simulink model "Adaptive_Cruise_Conrol_System"  (R2019a)
settings: Solver=VariableStepAuto  StartTime=0.0  StopTime=10.0  RelTol=1e-3
settings Model: Creator=賽維涅什  LastModifiedBy=賽維涅什

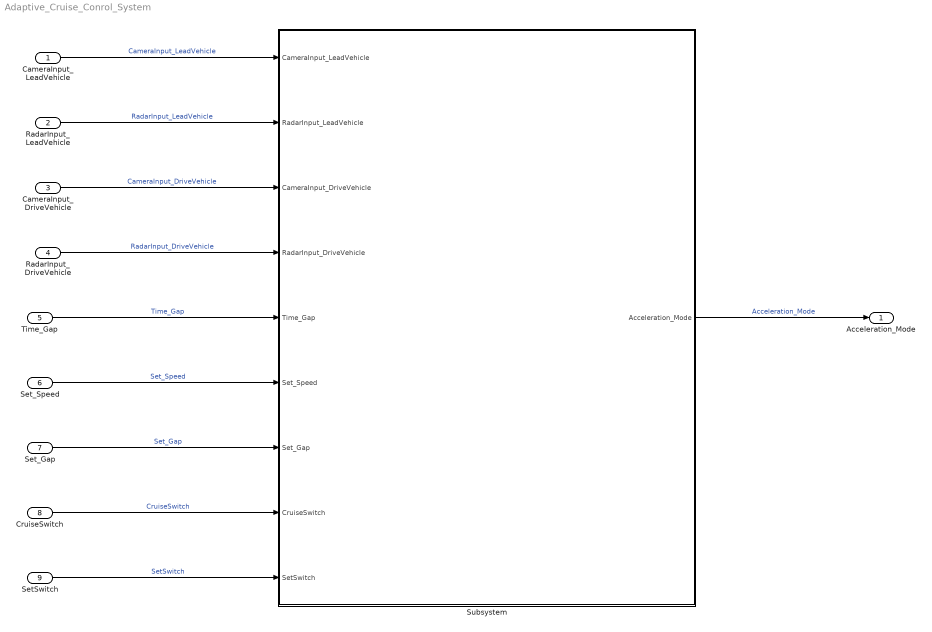
== system Adaptive_Cruise_Conrol_System ==
  CameraInput_LeadVehicle : Inport
  RadarInput_LeadVehicle : Inport  Port=2
  CameraInput_DriveVehicle : Inport  Port=3
  RadarInput_DriveVehicle : Inport  Port=4
  Time_Gap : Inport  Port=5
  Set_Speed : Inport  Port=6
  Set_Gap : Inport  Port=7
  CruiseSwitch : Inport  Port=8
  SetSwitch : Inport  Port=9
  Subsystem : Subsystem
  Acceleration_Mode : Outport
  wires:
  CameraInput_LeadVehicle/1 -> Subsystem/1(CameraInput_LeadVehicle)  "CameraInput_LeadVehicle"
  RadarInput_LeadVehicle/1 -> Subsystem/2(RadarInput_LeadVehicle)  "RadarInput_LeadVehicle"
  CameraInput_DriveVehicle/1 -> Subsystem/3(CameraInput_DriveVehicle)  "CameraInput_DriveVehicle"
  RadarInput_DriveVehicle/1 -> Subsystem/4(RadarInput_DriveVehicle)  "RadarInput_DriveVehicle"
  Time_Gap/1 -> Subsystem/5(Time_Gap)  "Time_Gap"
  Set_Speed/1 -> Subsystem/6(Set_Speed)  "Set_Speed"
  Set_Gap/1 -> Subsystem/7(Set_Gap)  "Set_Gap"
  CruiseSwitch/1 -> Subsystem/8(CruiseSwitch)  "CruiseSwitch"
  SetSwitch/1 -> Subsystem/9(SetSwitch)  "SetSwitch"
  Subsystem/1(Acceleration_Mode) -> Acceleration_Mode/1  "Acceleration_Mode"

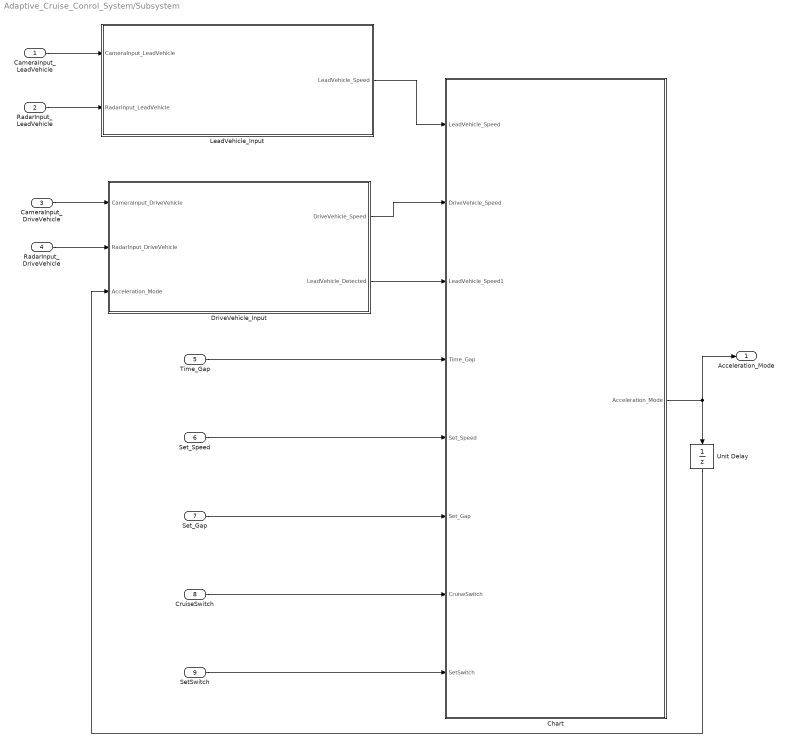
== system Adaptive_Cruise_Conrol_System/Subsystem ==
  CameraInput_LeadVehicle : Inport
  RadarInput_LeadVehicle : Inport  Port=2
  CameraInput_DriveVehicle : Inport  Port=3
  RadarInput_DriveVehicle : Inport  Port=4
  Time_Gap : Inport  Port=5
  Set_Speed : Inport  Port=6
  Set_Gap : Inport  Port=7
  CruiseSwitch : Inport  Port=8
  SetSwitch : Inport  Port=9
  Chart : Stateflow chart  BlockKeywords=__PRM__SERIALIZED__DATA__:Stateflow Chart,Stateflow Diagram  TreatAsAtomicUnit=on
  DriveVehicle_Input : Subsystem
  LeadVehicle_Input : Subsystem
  Unit Delay : UnitDelay  SampleTime=-1  HasFrameUpgradeWarning=on
  Acceleration_Mode : Outport
  wires:
  CameraInput_LeadVehicle/1 -> LeadVehicle_Input/1(CameraInput_LeadVehicle)
  DriveVehicle_Input/1(DriveVehicle_Speed) -> Chart/2(DriveVehicle_Speed)
  Chart/1(Acceleration_Mode) -> Acceleration_Mode/1, Unit Delay/1
  RadarInput_LeadVehicle/1 -> LeadVehicle_Input/2(RadarInput_LeadVehicle)
  Set_Speed/1 -> Chart/5(Set_Speed)
  Set_Gap/1 -> Chart/6(Set_Gap)
  CameraInput_DriveVehicle/1 -> DriveVehicle_Input/1(CameraInput_DriveVehicle)
  LeadVehicle_Input/1(LeadVehicle_Speed) -> Chart/1(LeadVehicle_Speed)
  Unit Delay/1 -> DriveVehicle_Input/3(Acceleration_Mode)
  CruiseSwitch/1 -> Chart/7(CruiseSwitch)
  Time_Gap/1 -> Chart/4(Time_Gap)
  DriveVehicle_Input/2(LeadVehicle_Detected) -> Chart/3(LeadVehicle_Speed1)
  RadarInput_DriveVehicle/1 -> DriveVehicle_Input/2(RadarInput_DriveVehicle)
  SetSwitch/1 -> Chart/8(SetSwitch)

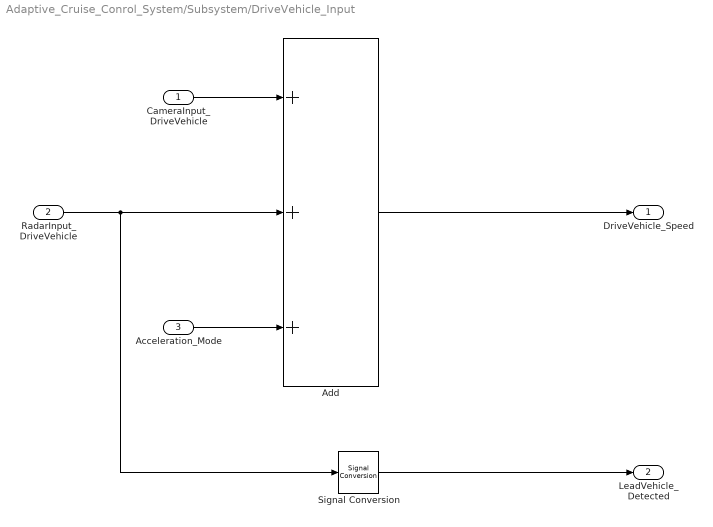
== system Adaptive_Cruise_Conrol_System/Subsystem/DriveVehicle_Input ==
  CameraInput_DriveVehicle : Inport
  RadarInput_DriveVehicle : Inport  Port=2
  Acceleration_Mode : Inport  Port=3
  Add : Sum  Inputs=+++
  Signal Conversion : SignalConversion  OverrideOpt=off
  DriveVehicle_Speed : Outport
  LeadVehicle_Detected : Outport  Port=2
  wires:
  CameraInput_DriveVehicle/1 -> Add/1
  RadarInput_DriveVehicle/1 -> Signal Conversion/1, Add/2
  Acceleration_Mode/1 -> Add/3
  Add/1 -> DriveVehicle_Speed/1
  Signal Conversion/1 -> LeadVehicle_Detected/1

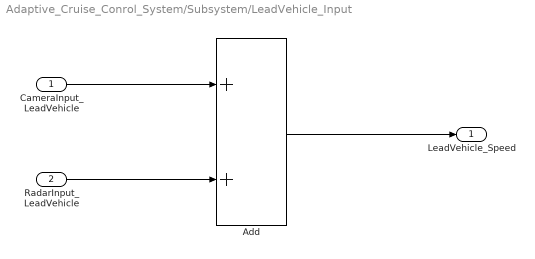
== system Adaptive_Cruise_Conrol_System/Subsystem/LeadVehicle_Input ==
  CameraInput_LeadVehicle : Inport
  RadarInput_LeadVehicle : Inport  Port=2
  Add : Sum
  LeadVehicle_Speed : Outport
  wires:
  CameraInput_LeadVehicle/1 -> Add/1
  RadarInput_LeadVehicle/1 -> Add/2
  Add/1 -> LeadVehicle_Speed/1

== stateflow chart Adaptive_Cruise_Conrol_System/Subsystem/Chart ==
  state ACC_ON_MODE
    en:Acceleration_Mode=1;
    state LeadVehicle_Detected_Follow
      en: Acceleration_Mode = 2;
    state LeadVehicle_Detected_Resume
      en: Acceleration_Mode = 3;
    state LeadVehicle_Not_Detected
      en: Acceleration_Mode = 1;
    state LeadVehicle_Speed_lessthan_set_Speed
      en: Acceleration_Mode = 4;
    state LeadVehicle_Not_Detected_Resume
      en: Acceleration_Mode = 1;
    state LeadVehicle_Speed_equal_Set_Speed
      en: Acceleration_Mode = 5;
    (default) -> LeadVehicle_Detected_Follow
    LeadVehicle_Detected_Follow -> LeadVehicle_Not_Detected [order 1] : [LeadVehicle_Detected == 0]
    LeadVehicle_Detected_Resume -> LeadVehicle_Detected_Follow [order 1] : [(DriveVehicle_Speed == Set_Speed)&&...
        | (LeadVehicle_Speed >= Set_Speed) &&...
        | (Time_Gap>= Set_Gap)]
    LeadVehicle_Detected_Resume -> LeadVehicle_Speed_equal_Set_Speed [order 2] : [(DriveVehicle_Speed<Set_Speed)&&...
        | (LeadVehicle_Speed > DriveVehicle_Speed)&&...
        | (Time_Gap >= Set_Gap)]
    LeadVehicle_Not_Detected -> LeadVehicle_Detected_Follow [order 1] : [(LeadVehicle_Detected == 1) &&...
        |  (DriveVehicle_Speed == Set_Speed) &&...
        | (LeadVehicle_Speed >= Set_Speed)&&...
        | (Time_Gap >= Set_Gap)]
    LeadVehicle_Speed_equal_Set_Speed -> LeadVehicle_Detected_Resume [order 2] : [(DriveVehicle_Speed<Set_Speed)&&...
        | (LeadVehicle_Speed>DriveVehicle_Speed)||...
        | (Time_Gap>=Set_Gap)]
    LeadVehicle_Detected_Follow -> LeadVehicle_Speed_lessthan_set_Speed [order 2] : [(LeadVehicle_Detected == 1) && ...
        | (LeadVehicle_Speed < Set_Speed)||...
        |  (Time_Gap< Set_Gap)]
    LeadVehicle_Not_Detected -> LeadVehicle_Speed_lessthan_set_Speed [order 2] : [(LeadVehicle_Detected == 1) &&...
        | (LeadVehicle_Speed < Set_Speed)||...
        | (Time_Gap < Set_Gap)]
    LeadVehicle_Speed_lessthan_set_Speed -> LeadVehicle_Not_Detected [order 1] : [(LeadVehicle_Detected == 0)&&...
        | (DriveVehicle_Speed == Set_Speed)]
    LeadVehicle_Speed_equal_Set_Speed -> LeadVehicle_Speed_lessthan_set_Speed [order 3] : [(LeadVehicle_Speed<Set_Speed)&&...
        | (LeadVehicle_Speed<DriveVehicle_Speed)||...
        | (Time_Gap==0.75*Set_Gap)]
    LeadVehicle_Speed_lessthan_set_Speed -> LeadVehicle_Speed_equal_Set_Speed [order 2] : [((LeadVehicle_Speed*1.25>=DriveVehicle_Speed)&&...
        | (LeadVehicle_Speed*0.75<=DriveVehicle_Speed))&&...
        | (DriveVehicle_Speed<Set_Speed)&&...
        | ((Time_Gap<=1.25*Set_Gap)&&...
        | (Time_Gap>=0.75*Set_Gap))]
    LeadVehicle_Speed_equal_Set_Speed -> LeadVehicle_Not_Detected_Resume [order 1] : [(LeadVehicle_Detected == 0)||...
        | (DriveVehicle_Speed <= Set_Speed)]
  state ACC_OFF_MODE
    en: Acceleration_Mode=0;
  state ACC_STANDBY_MODE
    en: Acceleration_Mode=1;
  (default) -> ACC_OFF_MODE
  ACC_ON_MODE -> ACC_OFF_MODE [order 2] : [CruiseSwitch==0]
  ACC_STANDBY_MODE -> ACC_OFF_MODE [order 2] : [CruiseSwitch == 0]
  ACC_OFF_MODE -> ACC_STANDBY_MODE : [CruiseSwitch == 1]
  ACC_ON_MODE -> ACC_STANDBY_MODE [order 1] : [SetSwitch == 0]
  ACC_STANDBY_MODE -> ACC_ON_MODE [order 1] : [SetSwitch == 1]
  data: LeadVehicle_Speed input; DriveVehicle_Speed input; LeadVehicle_Speed1 input; Time_Gap input; Set_Speed input; Set_Gap input; CruiseSwitch input; SetSwitch input; Acceleration_Mode output
